simulink model "PI_without_gain_scheduler"  (R2020a)
settings: Solver=VariableStepAuto  StartTime=0.0  StopTime=100  RelTol=1e-6  AbsTol=1e-6
settings Model: Creator=User  LastModifiedBy=User
settings SolverCC: AutoScaleAbsTol=off  ShapePreserveControl=EnableAll  ZeroCrossAlgorithm=Adaptive
settings DataIOCC: SaveOutput=off  SignalLogging=off  DSMLogging=off  SaveTime=off  ReturnWorkspaceOutputs=off

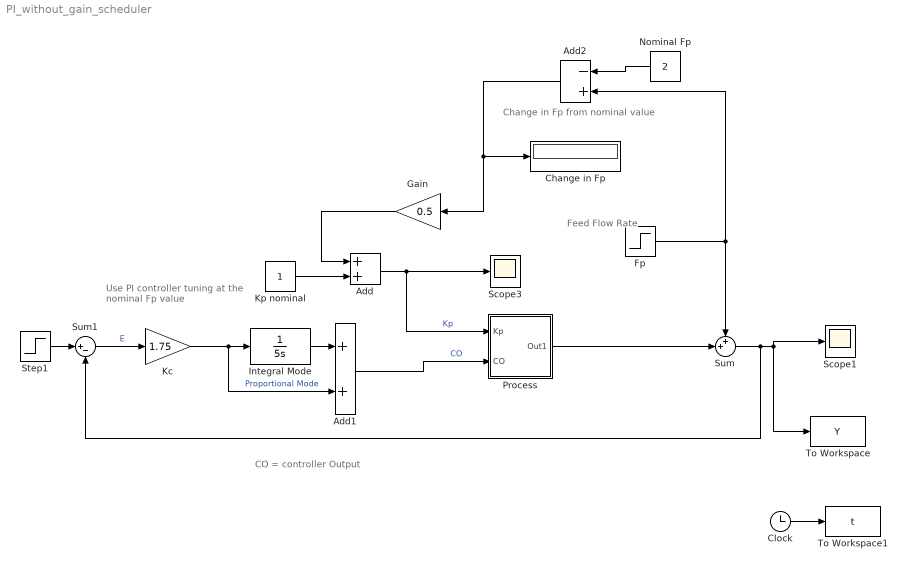
== system PI_without_gain_scheduler ==
  note: Use PI controller tuning
      | at the nominal Fp value
  note: CO = controller Output
  note: Change in Fp from nominal value
  note: Feed
      | Flow Rate
  Add : Sum
  Add1 : Sum
  Add2 : Sum  Inputs=-+
  Change in Fp : Display
  Clock : Clock
  Fp : Step  Time=0  Before=2  After=3  SampleTime=0
  Gain : Gain  Gain=0.5
  Integral Mode : TransferFcn  Denominator=[5 0]
  Kc : Gain  Gain=1.75
  Kp nominal : Constant
  Nominal Fp : Constant  Value=2
  Process : Subsystem
  Scope1 : Scope
  Scope3 : Scope
  Step1 : Step  Time=50  SampleTime=0
  Sum : Sum  Inputs=++|
  Sum1 : Sum  Inputs=|+-
  To Workspace : ToWorkspace  VariableName=Y  SampleTime=-1
  To Workspace1 : ToWorkspace  VariableName=t  SampleTime=-1
  wires:
  Sum/1 -> Sum1/2, To Workspace/1, Scope1/1
  Fp/1 -> Add2/2, Sum/1
  Kp nominal/1 -> Add/2
  Add/1 -> Process/1(Kp), Scope3/1  "Kp"
  Step1/1 -> Sum1/1
  Sum1/1 -> Kc/1  "E"
  Kc/1 -> Add1/2, Integral Mode/1  "Proportional Mode"
  Integral Mode/1 -> Add1/1
  Gain/1 -> Add/1
  Nominal Fp/1 -> Add2/1
  Add2/1 -> Gain/1, Change in Fp/1
  Clock/1 -> To Workspace1/1
  Add1/1 -> Process/2(CO)  "CO"
  Process/1(Out1) -> Sum/2

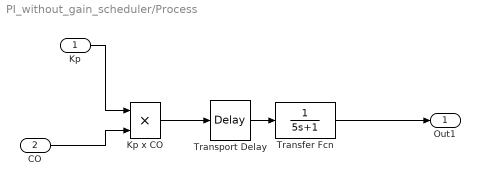
== system PI_without_gain_scheduler/Process ==
  Kp : Inport
  CO : Inport  Port=2
  Kp x CO : Product
  Transfer Fcn : TransferFcn  Denominator=[5 1]
  Transport Delay : TransportDelay  DelayTime=2
  Out1 : Outport
  wires:
  CO/1 -> Kp x CO/2
  Transport Delay/1 -> Transfer Fcn/1
  Kp/1 -> Kp x CO/1
  Kp x CO/1 -> Transport Delay/1
  Transfer Fcn/1 -> Out1/1
